simulink model "Moth_sim_v4"  (R2023b)
settings: Solver=ode4  StartTime=0.0  StopTime=inf  FixedStep=ST  RelTol=1e-3
values from neighbouring files (symbols this model uses):
  allpt = [G_sailor;AC_fw;AC_rudder;AC_sail]    [Moth_sim_start_v4.m]
  CD_sail = 0.05    [Moth_sim_start_v4.m]
  CL_sail = 0.4    [Moth_sim_start_v4.m]
  funCD_fw = polyfit(flap,cd_fw,3)    [Moth_sim_start_v4.m]
  funCD_r = polyfit(aoa,cd_r,2)    [Moth_sim_start_v4.m]
  funCL_fw = polyfit(flap,cl_fw,1)    [Moth_sim_start_v4.m]
  funCL_r = polyfit([0 aoa(end)],cl_r,1)    [Moth_sim_start_v4.m]
  funCM_fw = polyfit(flap,cm_fw,1)    [Moth_sim_start_v4.m]
  funCM_r = 0    [Moth_sim_start_v4.m]
  g = 9.81    [Moth_sim_start_v4.m]
  gamma_i = gamma_i*2*pi/360    (= -0.0872664625997)    [Moth_sim_start_v4.m]
  height_control = [ ... (first row only)    [Moth_sim_start_v4.m]
  I_yy_boat = I_yy_hull+I_yy_fw+I_yy_sail-50    (= 63)    [Moth_sim_start_v4.m]
  lower_z_limit = 0.10    (= 0.1)    [Moth_sim_start_v4.m]
  m_sailor = 75    [Moth_sim_start_v4.m]
  m_tot = m_sailor+m_boat    (= 110)    [Moth_sim_start_v4.m]
  mu = mu*2*pi/360    (= 0.523598775598)    [Moth_sim_start_v4.m]
  rho_air = 1.225    [Moth_sim_start_v4.m]
  rho_water = 998    [Moth_sim_start_v4.m]
  S_fw = 0.09    [Moth_sim_start_v4.m]
  S_r = 0.03946    [Moth_sim_start_v4.m]
  S_sail = 8.20    (= 8.2)    [Moth_sim_start_v4.m]
  ST = 0.01    [Moth_sim_start_v4.m]
  theta_i = theta_i*2*pi/360    (= 0.174532925199)    [Moth_sim_start_v4.m]
  TWA = TWA*2*pi/360    (= 1.57079632679)    [Moth_sim_start_v4.m]
  TWS = 7    [Moth_sim_start_v4.m]
  wand_attach_pos = mast_base+[1.05+0.5 0 -0.1]-G_hull    [Moth_sim_start_v4.m]
  wand_lenght = 1.25    [Moth_sim_start_v4.m]
  x_dot_i = 4    [Moth_sim_start_v4.m]
  z_i = -0.25    [Moth_sim_start_v4.m]
libraries: simulink x4, aerolibfltsims x2, aerolibanimutils x2, aerolibanim x1
settings Model: Creator=marco  LastModifiedBy=marco

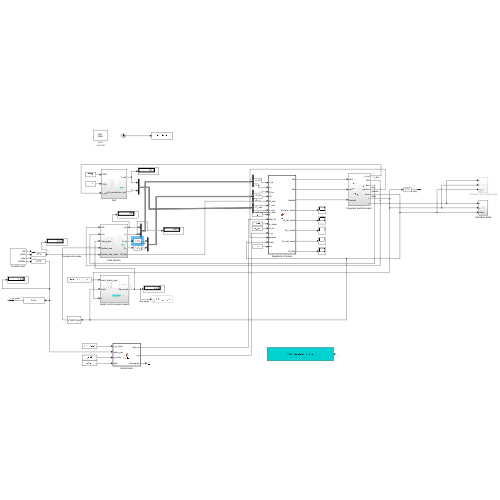
[thumbnail: Simulink's stored preview of the top-level diagram]
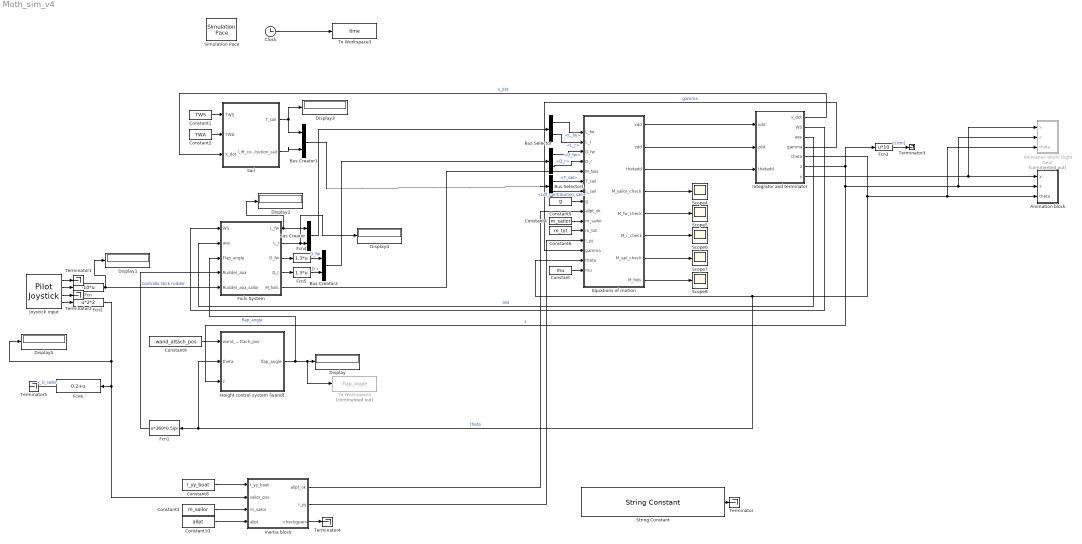
== system Moth_sim_v4 ==
  " " : BusSelector  OutputSignals=L_fw,L_r
  Animation block : Subsystem
  Animation block Flight Gear : Subsystem  Commented=on
  Bus Creator : BusCreator  Inputs=2
  Bus Creator1 : BusCreator  Inputs=2
  Bus Creator2 : BusCreator  Inputs=2
  Bus Selector : BusSelector  OutputSignals=D_fw,D_r
  Bus Selector1 : BusSelector  OutputSignals=T_sail,Lift_contribution_sail
  Clock : Clock
  Constant : Constant  Value=mu
  Constant1 : Constant  Value=TWS
  Constant10 : Constant  Value=allpt
  Constant2 : Constant  Value=TWA
  Constant3 : Constant  Value=m_sailor
  Constant4 : Constant  Value=m_sailor
  Constant5 : Constant  Value=g
  Constant6 : Constant  Value=m_tot
  Constant8 : Constant  Value=I_yy_boat
  Constant9 : Constant  Value=wand_attach_pos
  Display{,1..5} (6 alike) : Display
  Equations of motion : MATLAB Function  TreatAsAtomicUnit=on
  Fcn : Fcn  Expr=-10*u
  Fcn1 : Fcn  Expr=u*360*0.5/pi
  Fcn2 : Fcn  Expr=u*2*2
  Fcn3 : Fcn  Expr=u*10
  Fcn4 : Fcn  Expr=1.3*u
  Fcn5 : Fcn  Expr=1.3*u
  Fcn6 : Fcn  Expr=0.2+u
  Foils System : Subsystem
  Height control system (wand) : Subsystem
  Inertia block : MATLAB Function  TreatAsAtomicUnit=on
  Integrator and terminator : Subsystem
  Joystick input : aerolibanimutils/Pilot Joystick  JoystickID=Joystick1  OutputConfiguration=FourAxis  SampleTime=ST
  Sail : Subsystem
  Scope{4..8} (5 alike) : Scope
  Simulation Pace : aerolibanimutils/Simulation Pace  SimulationPace=1  SleepMode=Auto  OutputPaceError=off  SampleTime=ST
  String Constant : StringConstant  String='Made by Marco Salvato'
  Terminator{,1..5} (6 alike) : Terminator
  To Workspace1 : ToWorkspace  Commented=on  VariableName=flap_angle  SampleTime=-1
  To Workspace3 : ToWorkspace  VariableName=time  SampleTime=-1
  wires:
  Constant/1 -> Equations of motion/15(mu)
  Clock/1 -> To Workspace3/1
  Constant5/1 -> Equations of motion/8(g)
  Constant1/1 -> Sail/1(TWS)
  Constant2/1 -> Sail/2(TWA)
  Height control system (wand)/1(flap_angle) -> To Workspace1/1, Display/1, Foils System/3(Flap_angle)  "flap_angle"
  Constant6/1 -> Equations of motion/11(m_tot)
  Foils System/1(L_fw) -> Display2/1, Bus Creator/1
  Foils System/2(L_r) -> Display4/1, Bus Creator/2
  Bus Creator/1 -> " "/1
  " "/1 -> Equations of motion/1(L_fw)  "<L_fw>"
  " "/2 -> Equations of motion/2(L_r)  "<L_r>"
  Sail/1(T_sail) -> Display3/1, Bus Creator1/1
  Sail/2(Lift_contribution_sail) -> Bus Creator1/2
  Bus Creator1/1 -> Bus Selector1/1
  Bus Selector1/1 -> Equations of motion/6(T_sail)  "<T_sail>"
  Bus Selector1/2 -> Equations of motion/7(L_sail)  "<Lift_contribution_sail>"
  Constant4/1 -> Equations of motion/10(m_sailor)
  Foils System/5(M_foils) -> Equations of motion/5("M_foils ")
  Foils System/3(D_fw) -> Fcn4/1
  Foils System/4(D_r) -> Fcn5/1
  Bus Creator2/1 -> Bus Selector/1
  Bus Selector/1 -> Equations of motion/3(D_fw)  "<D_fw>"
  Bus Selector/2 -> Equations of motion/4(D_r)  "<D_r>"
  Fcn1/1 -> Foils System/4(Rudder_aoa)
  Fcn4/1 -> Bus Creator2/1  "D_fw"
  Fcn5/1 -> Bus Creator2/2  "D_r"
  Constant9/1 -> Height control system (wand)/1(wand_attach_pos)
  Constant8/1 -> Inertia block/1(I_yy_boat)
  Constant3/1 -> Inertia block/3(m_sailor)
  Constant10/1 -> Inertia block/4(allpt)
  Fcn2/1 -> Display5/1, Fcn6/1, Inertia block/2(sailor_pos)
  Inertia block/1(allpt_ok) -> Equations of motion/9(allpt_ok)
  Inertia block/2(I_yy) -> Equations of motion/12(I_yy)
  Integrator and terminator/5(theta) -> Animation block/3(theta), Animation block Flight Gear/3(theta), Equations of motion/14(theta), Height control system (wand)/2(theta), Fcn1/1  "theta"
  Equations of motion/1(xdd) -> Integrator and terminator/1(xdd)
  Equations of motion/2(zdd) -> Integrator and terminator/2(zdd)
  Equations of motion/3(thetadd) -> Integrator and terminator/3(thetadd)
  Integrator and terminator/1(x_dot) -> Sail/3(x_dot)  "x_dot"
  Integrator and terminator/2(WS) -> Foils System/1(WS)
  Integrator and terminator/3(aoa) -> Foils System/2(aoa)  "aoa"
  Integrator and terminator/4(gamma) -> Equations of motion/13(gamma)  "gamma"
  Equations of motion/5(M_fw_check) -> Scope5/1
  Equations of motion/4(M_sailor_check) -> Scope4/1
  Equations of motion/6(M_r_check) -> Scope6/1
  Equations of motion/7(M_sail_check) -> Scope7/1
  Equations of motion/8(M_foils) -> Scope8/1
  Integrator and terminator/7(x) -> Animation block Flight Gear/1(x), Animation block/1(x)
  String Constant/1 -> Terminator/1
  Integrator and terminator/6(z) -> Fcn3/1, Animation block/2(z), Animation block Flight Gear/2(z), Height control system (wand)/3(z)  "z"
  Fcn/1 -> Display1/1, Foils System/5(Rudder_aoa_sailor)  "Controllo stick rudder"
  Joystick input/2 -> Fcn/1
  Joystick input/4 -> Fcn2/1
  Joystick input/1 -> Terminator1/1
  Joystick input/3 -> Terminator2/1
  Fcn3/1 -> Terminator3/1  "z [dm]"
  Inertia block/3(checkgpers) -> Terminator4/1
  Fcn6/1 -> Terminator5/1  "x_G_sailor"

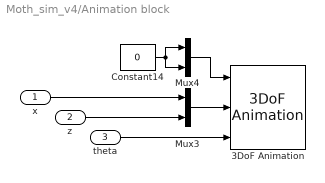
== system Moth_sim_v4/Animation block ==
  x : Inport
  z : Inport  Port=2
  theta : Inport  Port=3
  3DoF Animation : aerolibanim/3DoF Animation  u1=[0 10000 -20 20 -20 0]  u2=ST  u3=0.031  u5=Fly alongside  u6=[0 20 0]  u7=8  u8=on
  Constant14 : Constant  Value=0
  Mux3 : Mux  Inputs=2
  Mux4 : Mux  Inputs=2
  wires:
  Constant14/1 -> Mux4/1, Mux4/2
  Mux4/1 -> 3DoF Animation/1
  theta/1 -> 3DoF Animation/3
  Mux3/1 -> 3DoF Animation/2
  z/1 -> Mux3/2
  x/1 -> Mux3/1

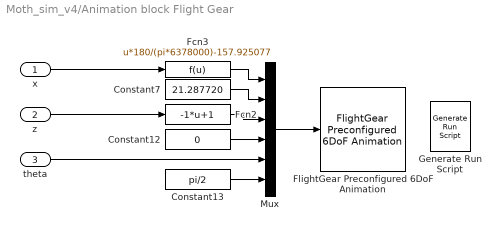
== system Moth_sim_v4/Animation block Flight Gear ==
  x : Inport
  z : Inport  Port=2
  theta : Inport  Port=3
  Constant12 : Constant  Value=0
  Constant13 : Constant  Value=pi/2
  Constant7 : Constant  Value=21.287720
  Fcn2 : Fcn  Expr=-1*u+1
  Fcn3 : Fcn  Expr=u*180/(pi*6378000)-157.925077
  FlightGear Preconfigured 6DoF Animation : aerolibfltsims/FlightGear Preconfigured 6DoF Animation  xFlightGearVersion=v2019.1  DestinationIpAddress=127.0.0.1  DestinationPort=5502  SampleTime=ST  packetVersion=24
  Generate Run Script : aerolibfltsims/Generate Run Script  Architecture=Win64  dataFlow=Send  GeometryModelName=c172p  AirportId=VCE  RunwayId=10L  InitialAltitude=7224  InitialHeading=113  OffsetDistance=4.72  OffsetAzimuth=0  InstallScenery=off  DisableShaders=on  OriginAddress=127.0.0.1  DestinationPort=5502  OriginPort=5505  LocalAddress=127.0.0.1  OutputFileName=runfg.bat  FlightGearBaseDirectory=C:\Program Files\FlightGear 2020.3
  Mux : Mux  Inputs=6
  wires:
  z/1 -> Fcn2/1
  theta/1 -> Mux/5
  Constant7/1 -> Mux/2
  Fcn3/1 -> Mux/1
  Fcn2/1 -> Mux/3
  Mux/1 -> FlightGear Preconfigured 6DoF Animation/1
  Constant12/1 -> Mux/4
  Constant13/1 -> Mux/6
  x/1 -> Fcn3/1

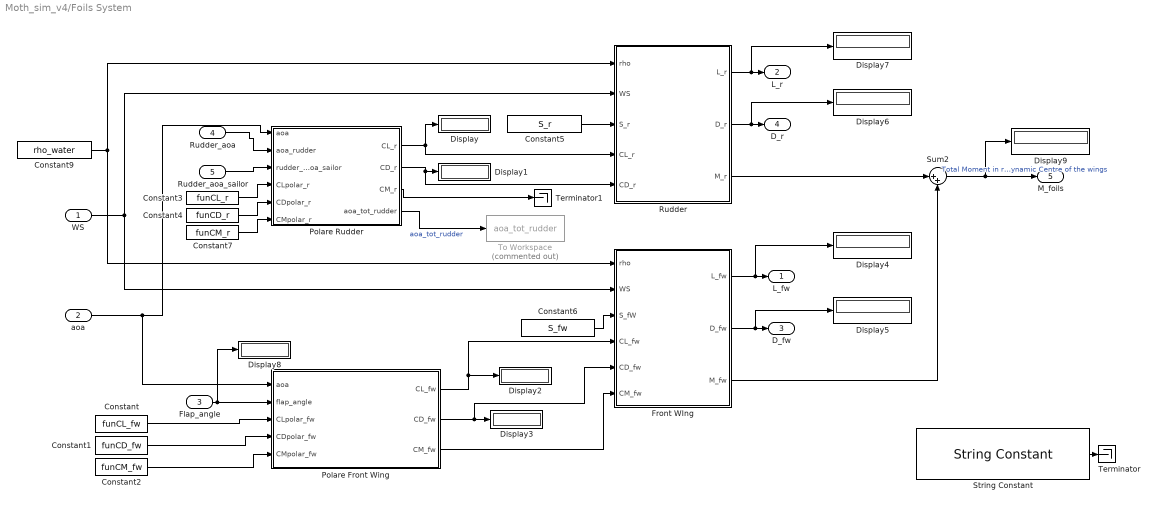
== system Moth_sim_v4/Foils System ==
  WS : Inport
  aoa : Inport  Port=2
  Flap_angle : Inport  Port=3
  Rudder_aoa : Inport  Port=4
  Rudder_aoa_sailor : Inport  Port=5
  Constant : Constant  Value=funCL_fw
  Constant1 : Constant  Value=funCD_fw
  Constant2 : Constant  Value=funCM_fw
  Constant3 : Constant  Value=funCL_r
  Constant4 : Constant  Value=funCD_r
  Constant5 : Constant  Value=S_r
  Constant6 : Constant  Value=S_fw
  Constant7 : Constant  Value=funCM_r
  Constant9 : Constant  Value=rho_water
  Display{,1..9} (10 alike) : Display
  Front WIng : MATLAB Function  TreatAsAtomicUnit=on
  Polare Front Wing : MATLAB Function  TreatAsAtomicUnit=on
  Polare Rudder : MATLAB Function  TreatAsAtomicUnit=on
  Rudder : MATLAB Function  TreatAsAtomicUnit=on
  String Constant : StringConstant  String='Made by Marco Salvato'
  Sum2 : Sum  Inputs=|++
  Terminator : Terminator
  Terminator1 : Terminator
  To Workspace : ToWorkspace  Commented=on  VariableName=aoa_tot_rudder  SaveFormat=Timeseries  SampleTime=-1
  L_fw : Outport
  L_r : Outport  Port=2
  D_fw : Outport  Port=3
  D_r : Outport  Port=4
  M_foils : Outport  Port=5
  wires:
  WS/1 -> Front WIng/2(WS), Rudder/2(WS)
  Constant9/1 -> Rudder/1(rho), Front WIng/1(rho)
  Constant5/1 -> Rudder/3(S_r)
  Constant6/1 -> Front WIng/3(S_fW)
  Rudder/3(M_r) -> Sum2/1
  Front WIng/3(M_fw) -> Sum2/2
  Sum2/1 -> Display9/1, M_foils/1  "Total Moment in respect to Aerodynamic Centre of the wings"
  Flap_angle/1 -> Display8/1, Polare Front Wing/2(flap_angle)
  Polare Front Wing/1(CL_fw) -> Display2/1, Front WIng/4(CL_fw)
  Polare Front Wing/2(CD_fw) -> Front WIng/5(CD_fw), Display3/1
  Polare Front Wing/3(CM_fw) -> Front WIng/6(CM_fw)
  Constant/1 -> Polare Front Wing/3(CLpolar_fw)
  Constant1/1 -> Polare Front Wing/4(CDpolar_fw)
  Constant2/1 -> Polare Front Wing/5(CMpolar_fw)
  Rudder_aoa/1 -> Polare Rudder/2(aoa_rudder)
  Polare Rudder/1(CL_r) -> Display/1, Rudder/4(CL_r)
  Polare Rudder/2(CD_r) -> Rudder/5(CD_r), Display1/1
  Polare Rudder/3(CM_r) -> Terminator1/1
  Constant3/1 -> Polare Rudder/4(CLpolar_r)
  Constant4/1 -> Polare Rudder/5(CDpolar_r)
  Front WIng/1(L_fw) -> Display4/1, L_fw/1
  Rudder/1(L_r) -> Display7/1, L_r/1
  Front WIng/2(D_fw) -> Display5/1, D_fw/1
  Rudder/2(D_r) -> Display6/1, D_r/1
  aoa/1 -> Polare Front Wing/1(aoa), Polare Rudder/1(aoa)
  Constant7/1 -> Polare Rudder/6(CMpolar_r)
  Rudder_aoa_sailor/1 -> Polare Rudder/3(rudder_aoa_sailor)
  Polare Rudder/4(aoa_tot_rudder) -> To Workspace/1  "aoa_tot_rudder"
  String Constant/1 -> Terminator/1

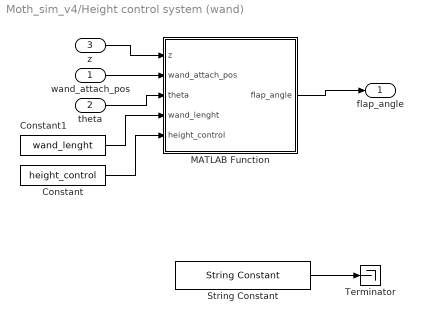
== system Moth_sim_v4/Height control system (wand) ==
  wand_attach_pos : Inport
  theta : Inport  Port=2
  z : Inport  Port=3
  Constant : Constant  Value=height_control  VectorParams1D=off
  Constant1 : Constant  Value=wand_lenght
  MATLAB Function : MATLAB Function  TreatAsAtomicUnit=on
  String Constant : StringConstant  String='Made by Marco Salvato'
  Terminator : Terminator
  flap_angle : Outport
  wires:
  Constant/1 -> MATLAB Function/5(height_control)
  z/1 -> MATLAB Function/1(z)
  Constant1/1 -> MATLAB Function/4(wand_lenght)
  MATLAB Function/1(flap_angle) -> flap_angle/1
  wand_attach_pos/1 -> MATLAB Function/2(wand_attach_pos)
  theta/1 -> MATLAB Function/3(theta)
  String Constant/1 -> Terminator/1

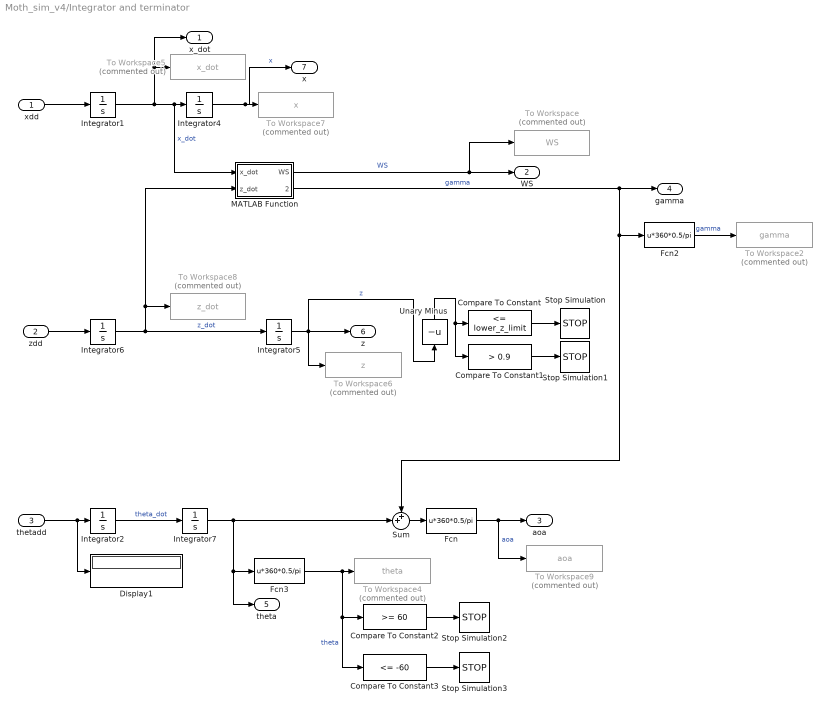
== system Moth_sim_v4/Integrator and terminator ==
  xdd : Inport
  zdd : Inport  Port=2
  thetadd : Inport  Port=3
  Compare To Constant : simulink/Logic and Bit Operations/Compare To Constant  relop=<=  const=lower_z_limit  OutDataTypeStr=boolean
  Compare To Constant1 : simulink/Logic and Bit Operations/Compare To Constant  relop=>  const=0.9  OutDataTypeStr=boolean
  Compare To Constant2 : simulink/Logic and Bit Operations/Compare To Constant  relop=>=  const=60  OutDataTypeStr=boolean
  Compare To Constant3 : simulink/Logic and Bit Operations/Compare To Constant  relop=<=  const=-60  OutDataTypeStr=boolean
  Display1 : Display
  Fcn : Fcn  Expr=u*360*0.5/pi
  Fcn2 : Fcn  Expr=u*360*0.5/pi
  Fcn3 : Fcn  Expr=u*360*0.5/pi
  Integrator1 : Integrator  InitialCondition=x_dot_i
  Integrator2 : Integrator
  Integrator4 : Integrator
  Integrator5 : Integrator  InitialCondition=z_i
  Integrator6 : Integrator  InitialCondition=x_dot_i*tan(gamma_i)
  Integrator7 : Integrator  InitialCondition=theta_i
  MATLAB Function : MATLAB Function  TreatAsAtomicUnit=on
  Stop Simulation{,1..3} (4 alike) : Stop
  Sum : Sum  Inputs=++|
  To Workspace : ToWorkspace  Commented=on  VariableName=WS  SampleTime=-1
  To Workspace2 : ToWorkspace  Commented=on  VariableName=gamma  SampleTime=-1
  To Workspace4 : ToWorkspace  Commented=on  VariableName=theta  SampleTime=-1
  To Workspace5 : ToWorkspace  Commented=on  VariableName=x_dot  SampleTime=-1
  To Workspace6 : ToWorkspace  Commented=on  VariableName=z  SampleTime=-1
  To Workspace7 : ToWorkspace  Commented=on  VariableName=x  SampleTime=-1
  To Workspace8 : ToWorkspace  Commented=on  VariableName=z_dot  SampleTime=-1
  To Workspace9 : ToWorkspace  Commented=on  VariableName=aoa  SampleTime=-1
  Unary Minus : UnaryMinus
  x_dot : Outport
  WS : Outport  Port=2
  aoa : Outport  Port=3
  gamma : Outport  Port=4
  theta : Outport  Port=5
  z : Outport  Port=6
  x : Outport  Port=7
  wires:
  Unary Minus/1 -> Compare To Constant1/1, Compare To Constant/1
  MATLAB Function/2(gamma) -> Sum/1, Fcn2/1, gamma/1  "gamma"
  Integrator5/1 -> To Workspace6/1, z/1, Unary Minus/1  "z"
  MATLAB Function/1(WS) -> To Workspace/1, WS/1  "WS"
  Compare To Constant1/1 -> Stop Simulation1/1
  thetadd/1 -> Display1/1, Integrator2/1
  Integrator6/1 -> Integrator5/1, MATLAB Function/2(z_dot), To Workspace8/1  "z_dot"
  Integrator7/1 -> Fcn3/1, theta/1, Sum/2
  zdd/1 -> Integrator6/1
  Integrator4/1 -> To Workspace7/1, x/1  "x"
  Fcn3/1 -> Compare To Constant3/1, Compare To Constant2/1, To Workspace4/1  "theta"
  Sum/1 -> Fcn/1
  Integrator2/1 -> Integrator7/1  "theta_dot"
  Integrator1/1 -> x_dot/1, To Workspace5/1, MATLAB Function/1(x_dot), Integrator4/1  "x_dot"
  Compare To Constant/1 -> Stop Simulation/1
  Fcn2/1 -> To Workspace2/1  "gamma"
  Fcn/1 -> To Workspace9/1, aoa/1  "aoa"
  xdd/1 -> Integrator1/1
  Compare To Constant2/1 -> Stop Simulation2/1
  Compare To Constant3/1 -> Stop Simulation3/1

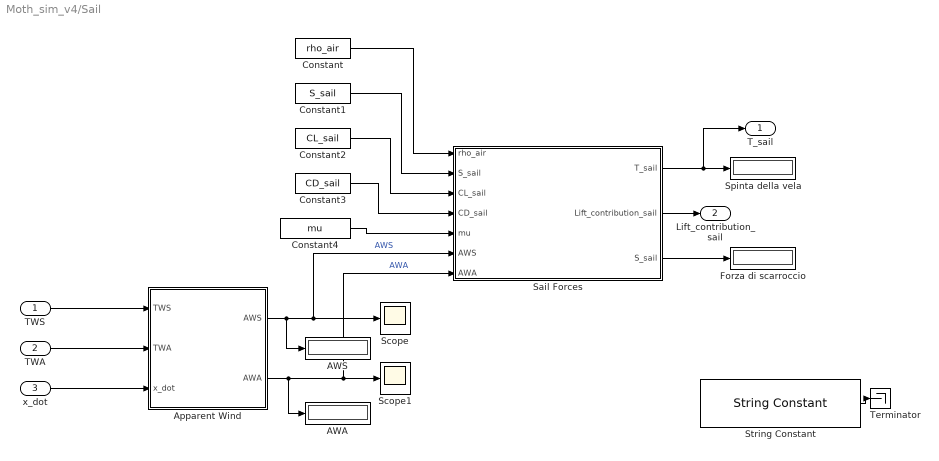
== system Moth_sim_v4/Sail ==
  TWS : Inport
  TWA : Inport  Port=2
  x_dot : Inport  Port=3
  AWA : Display
  AWS : Display
  Apparent Wind : MATLAB Function  TreatAsAtomicUnit=on
  Constant : Constant  Value=rho_air
  Constant1 : Constant  Value=S_sail
  Constant2 : Constant  Value=CL_sail
  Constant3 : Constant  Value=CD_sail
  Constant4 : Constant  Value=mu
  Forza di scarroccio : Display
  Sail Forces : MATLAB Function  TreatAsAtomicUnit=on
  Scope : Scope
  Scope1 : Scope
  Spinta della vela : Display
  String Constant : StringConstant  String='Made by Marco Salvato'
  Terminator : Terminator
  T_sail : Outport
  Lift_contribution_sail : Outport  Port=2
  wires:
  TWS/1 -> Apparent Wind/1(TWS)
  TWA/1 -> Apparent Wind/2(TWA)
  x_dot/1 -> Apparent Wind/3(x_dot)
  Apparent Wind/1(AWS) -> AWS/1, Scope/1, Sail Forces/6(AWS)  "AWS"
  Apparent Wind/2(AWA) -> Scope1/1, Sail Forces/7(AWA), AWA/1  "AWA"
  Sail Forces/3(S_sail) -> Forza di scarroccio/1
  Constant/1 -> Sail Forces/1(rho_air)
  Constant1/1 -> Sail Forces/2("S_sail ")
  Constant3/1 -> Sail Forces/4(CD_sail)
  Constant2/1 -> Sail Forces/3(CL_sail)
  Sail Forces/1(T_sail) -> T_sail/1, Spinta della vela/1
  Constant4/1 -> Sail Forces/5(mu)
  Sail Forces/2(Lift_contribution_sail) -> Lift_contribution_sail/1
  String Constant/1 -> Terminator/1

== matlab function Moth_sim_v4/Sail/Sail Forces ==
  data: rho_air input; S_sail input; CL_sail input; CD_sail input; mu input; AWS input; T_sail output; Lift_contribution_sail output; AWA input; S_sail output
function [T_sail,Lift_contribution_sail,S_sail] = sailforces(rho_air,S_sail,CL_sail,CD_sail,mu,AWS,AWA)

% T=forza di spinta della vela nella direzione longitudinale della barca
% (rotta)
% S=forza di scarroccio nella direzione trasversale della barca

% Si suppone che la vela venga mantenuta ad un AOA costante rispetto ad AWA
% ("se il velista è bravo"). L'AOA a cui viene mantenuta è quello di
% massima efficienza della vela, ovvero dai 4 ai 6 gradi

% Da XFLR, si calcola che la vela con un angolo dai 4 ai 6 gradi ha un CL
% medio pari a CL_sail=0.17 e un CD_sail=0.01

L_sail=0.5*rho_air*AWS^2*S_sail*CL_sail;
D_sail=0.5*rho_air*AWS^2*S_sail*CD_sail;

AWA=AWA*2*pi/360;
T_sail=(L_sail*cos(mu))*sin(AWA)-(D_sail*cos(mu))*cos(AWA);
S_sail=(L_sail*cos(mu))*cos(AWA)+(D_sail*cos(mu))*sin(AWA);

Lift_contribution_sail=L_sail*tan(mu)+D_sail*tan(mu);
% NB T_sail include già il drag dovuto alla vela in direzione longitudinale

== matlab function Moth_sim_v4/Height control system (wand)/MATLAB Function ==
  data: z input; wand_attach_pos input; theta input; flap_angle output; wand_lenght input; height_control input
function flap_angle = flapangle(z,wand_attach_pos,theta,wand_lenght,height_control)

p=polyfit(height_control(:,1),height_control(:,2),2);
z_wand=-z+wand_attach_pos(1)*sin(theta)+wand_attach_pos(3)*cos(theta);
flap_angle=polyval(p,z_wand);

== matlab function Moth_sim_v4/Foils System/Polare Front Wing ==
  data: aoa input; flap_angle input; CLpolar_fw input; CDpolar_fw input; CMpolar_fw input; CL_fw output; CD_fw output; CM_fw output
function [CL_fw,CD_fw,CM_fw]=polar_frontwing(aoa,flap_angle,CLpolar_fw,CDpolar_fw,CMpolar_fw)

CL_fw=polyval(CLpolar_fw,aoa+flap_angle);
CD_fw=polyval(CDpolar_fw,aoa+flap_angle);
CM_fw=polyval(CMpolar_fw,aoa+flap_angle);

== matlab function Moth_sim_v4/Foils System/Polare Rudder ==
  data: aoa input; aoa_rudder input; rudder_aoa_sailor input; CL_r output; CD_r output; CM_r output; CLpolar_r input; CDpolar_r input; CMpolar_r input; aoa_tot_rudder output
function [CL_r,CD_r,CM_r,aoa_tot_rudder] = polar_rudder(aoa,aoa_rudder,rudder_aoa_sailor, CLpolar_r,CDpolar_r,CMpolar_r)

% CL_r=polyval(CLpolar_r,aoa+aoa_rudder*1.3+rudder_aoa_sailor);
% CD_r=polyval(CDpolar_r,aoa+aoa_rudder*1.3+rudder_aoa_sailor);
% CM_r=polyval(CMpolar_r,aoa+aoa_rudder*1.3+rudder_aoa_sailor);
%aoa_tot_rudder=aoa+aoa_rudder*1.3+rudder_aoa_sailor;

CL_r=polyval(CLpolar_r,aoa+rudder_aoa_sailor);
CD_r=polyval(CDpolar_r,aoa+rudder_aoa_sailor);
CM_r=polyval(CMpolar_r,aoa+rudder_aoa_sailor);

aoa_tot_rudder=aoa+rudder_aoa_sailor;

% NB: al momento aoa_rudder non è usato perchè sarebbe un controllo
% automatico forzato del timone. tutto il controllo è lasciato al timoniere

== matlab function Moth_sim_v4/Integrator and terminator/MATLAB Function ==
  data: WS output; x_dot input; gamma output; z_dot input
function [WS,gamma] = gamma(x_dot,z_dot)

WS=sqrt(x_dot^2+z_dot^2);
gamma=atan(z_dot/x_dot);

== matlab function Moth_sim_v4/Inertia block ==
  data: I_yy_boat input; sailor_pos input; allpt_ok output; m_sailor input; allpt input; I_yy output; checkgpers output
function [allpt_ok,I_yy,checkgpers] = inertia(I_yy_boat,sailor_pos,m_sailor,allpt)

allpt_ok=allpt;
allpt_ok(1,1)=allpt_ok(1,1)+sailor_pos;
checkgpers=allpt_ok(1,1);
I_yy=I_yy_boat+m_sailor*norm(allpt_ok(1,:))^2;

== matlab function Moth_sim_v4/Sail/Apparent Wind ==
  data: TWS input; AWS output; TWA input; x_dot input; AWA output
function [AWS,AWA] = apparentwind(TWS,TWA,x_dot)

AWS_longitudinal=TWS*cos(TWA)+x_dot;
AWS_transveral=TWS*sin(TWA);
AWS=sqrt(AWS_longitudinal^2+AWS_transveral^2);
AWA=atan(AWS_transveral/AWS_longitudinal)*360*0.5/pi;

== matlab function Moth_sim_v4/Equations of motion ==
  data: L_fw input; L_r input; D_fw input; D_r input; M_foils input; T_sail input; L_sail input; g input; allpt_ok input; m_sailor input; m_tot input; I_yy input; gamma input; theta input; mu input; xdd output; zdd output; thetadd output; M_sailor_check output; M_fw_check output; M_r_check output; M_sail_check output; M_foils output
function [xdd,zdd,thetadd,M_sailor_check,M_fw_check,M_r_check,M_sail_check,M_foils] = eqs(L_fw,L_r,D_fw,D_r,M_foils,T_sail,L_sail,g,allpt_ok,m_sailor,m_tot,I_yy,gamma,theta,mu)

% Vettori forze
L_fw_vect=[0,0,-L_fw]'; % Rispetto a SDR WS
D_fw_vect=[-D_fw,0,0]'; % Rispetto a SDR WS
L_r_vect=[0,0,-L_r]'; % Rispetto a SDR WS
D_r_vect=[-D_r,0,0]'; % Rispetto a SDR WS
T_sail_vect=[T_sail,0,0]'; % Rispetto a SDR I
L_sail_vect=[0,0,-L_sail]'; % Rispetto a SDR I
g_vect=[0,0,g]'; % Rispetto a SDR I

% Matrice di rotazione tra i SDR
ROT_WS_to_I=[cos(gamma),0,-sin(gamma);0,0,0;sin(gamma),0,cos(gamma)];
ROT_I_to_Body=[cos(theta),0,-sin(theta);0,0,0;sin(theta),0,cos(theta)];
ROT_WS_to_Body=ROT_I_to_Body*ROT_WS_to_I;



% Equazione traslazionale (rispetto a SDR I)
% trasl_acc=(ROT_WS_to_I*(L_fw_vect+L_r_vect+D_fw_vect+D_r_vect)+T_sail_vect+L_sail_vect+m_tot*g_vect)/m_tot;
% xdd=trasl_acc(1);
% zdd=trasl_acc(3);

xdd=((L_fw+L_r)*sin(gamma)-(D_fw+D_r)*cos(gamma)+T_sail)/m_tot;
zdd=(-(L_fw+L_r)*cos(gamma)*cos(mu)-(D_fw+D_r)*sin(gamma)*cos(mu)-L_sail*cos(mu)+m_tot*g)/m_tot;



% Equazione rotazionale (rispetto a SDR Body)

thetadd3d=(cross(allpt_ok(1,:)',ROT_I_to_Body*g_vect*m_sailor)+... % M_sailor
    cross(allpt_ok(2,:)',ROT_WS_to_Body*(L_fw_vect+D_fw_vect))+... % M_fw
    cross(allpt_ok(3,:)',ROT_WS_to_Body*(L_r_vect+D_r_vect))+... % M_r
    cross(allpt_ok(4,:)',ROT_I_to_Body*(T_sail_vect+L_sail_vect))+... M_sail
    [0;M_foils;0])*cos(mu)/I_yy; % M_foils (rispetto al AC)
thetadd=thetadd3d(2);

% Calcolo dei momenti generati dai vari elementi rispetto al CM_hull solo per un controllo 
M_sailor_check=cross(allpt_ok(1,:)',ROT_I_to_Body*g_vect*m_sailor);
M_fw_check=cross(allpt_ok(2,:)',ROT_WS_to_Body*(L_fw_vect+D_fw_vect));
M_r_check=cross(allpt_ok(3,:)',ROT_WS_to_Body*(L_r_vect+D_r_vect));
M_sail_check=cross(allpt_ok(4,:)',ROT_I_to_Body*(T_sail_vect+L_sail_vect));
M_foils;

% thetadd=(abs(allpt(1,1))*g*m_sailor*cos(theta)+... % sailore
%     abs(allpt(1,3))*g*m_sailor*sin(theta)+...
%     abs(allpt(2,1))*L_fw*cos(theta+gamma)+...
%     abs(allpt(2,3))*L_fw*sin(theta+gamma)+...
%     abs(allpt(2,1))*D_fw*sin(theta+gamma)+...
%     -abs(allpt(2,3))*D_fw*cos(theta+gamma)+... % fine FW
%     -abs(allpt(3,1))*L_r*cos(theta+gamma)+...
%     -abs(allpt(3,3))*L_r*sin(theta+gamma)+...
%     -abs(allpt(3,1))*D_r*sin(theta+gamma)+...
%     -abs(allpt(3,3))*D_r*cos(theta+gamma)+... % fine Rudder
%     -abs(allpt(4,1))*T_sail*cos(theta)+...
%     abs(allpt(4,1))*T_sail*sin(theta)+...  % fine vela
%     -M_foils)*cos(mu)/I_yy;
% 

%% Made by Marco Salvato

== matlab function Moth_sim_v4/Foils System/Rudder ==
  data: rho input; WS input; S_r input; L_r output; D_r output; M_r output; CL_r input; CD_r input
function [L_r,D_r,M_r]=rudder(rho,WS,S_r,CL_r,CD_r)

L_r=0.5*rho*WS^2*S_r*CL_r;
D_r=0.5*rho*WS^2*S_r*CD_r;
M_r=0;

== matlab function Moth_sim_v4/Foils System/Front WIng ==
  data: rho input; WS input; S_fW input; L_fw output; D_fw output; M_fw output; CL_fw input; CD_fw input; CM_fw input
function [L_fw,D_fw,M_fw]=frontwing(rho,WS,S_fW,CL_fw,CD_fw,CM_fw)

L_fw=0.5*rho*WS^2*S_fW*CL_fw;
D_fw=0.5*rho*WS^2*S_fW*CD_fw;
M_fw=0.5*rho*WS^2*S_fW*0.096*CM_fw; % 0.096 sta per la corda media che non avevo voglia di importare
